simulink model "FPRHX_Demo"  (R2023a)
settings: Solver=FixedStepAuto  StartTime=0.0  StopTime=259200  FixedStep=10  RelTol=1e-3
settings Model: Creator=Owner  LastModifiedBy=Owner

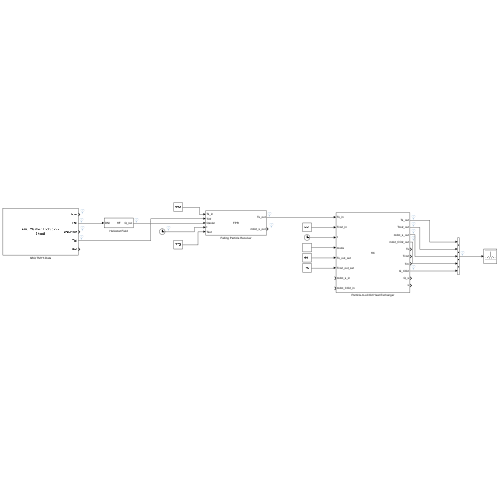
[thumbnail: Simulink's stored preview of the top-level diagram]
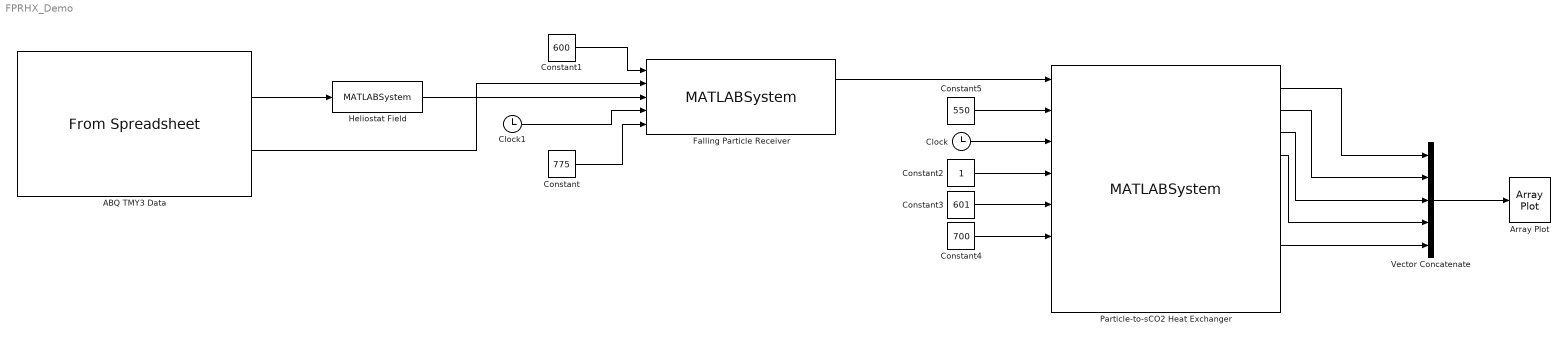
== system FPRHX_Demo ==
  ABQ TMY3 Data : FromSpreadsheet  FileName=ABQ_Weather_Lookup.xlsx  OutDataTypeStr=double
  Array Plot : ArrayPlot  WindowPosition=[1014.000000,178.000000,800.000000,500.000000,]  ScopeFrameLocation=window  YLimits=[-2854873.1962,317687.6016]
  Clock : Clock
  Clock1 : Clock
  Constant : Constant  Value=775
  Constant1 : Constant  Value=600
  Constant2 : Constant  OutDataTypeStr=boolean
  Constant3 : Constant  Value=601
  Constant4 : Constant  Value=700
  Constant5 : Constant  Value=550
  Falling Particle Receiver : MATLABSystem  System=FPR  H=1.2  W=1.2  d=0.0417  SimulateUsing=Code generation  Ts0=600  hInf=5  cp_s=1250  rho_s=3500  phi_s=0.6  epsilon_s=0.88  alpha_s=0.92  tauLag=1500  tauLead=100
      mask Type: FPR
      mask Display:
      | disp('FPR');
      | port_label('input',1,'Ts_in');
      | port_label('input',2,'Tinf');
      | port_label('input',3,'Qsolar');
      | port_label('input',4,'t');
      | port_label('input',5,'Tset');
      | port_label('output',1,'Ts_out');
      | port_label('output',2,'mdot_s_out');
  Heliostat Field : MATLABSystem  System=HF  n=150  H=5  W=5  eta_op=0.6  SimulateUsing=Code generation
      mask Type: HF
      mask Display:
      | disp('HF');
      | port_label('input',1,'DNI');
      | port_label('output',1,'Q_rec');
  Particle-to-sCO2 Heat Exchanger : MATLABSystem  System=HX  n=20  t_s=0.006  t_CO2=0.001  t_m=0.003  H=1.5  W=0.6  N_plate=33  SimulateUsing=Code generation  Ts0=600  Tco20=600  Tm0=25  h_s=450  h_CO2=3000  cp_s=1250  rho_s=3500  phi_s=0.6  cp_CO2=1250  rho_CO2=110  cp_m=500  rho_m=8000
      mask Type: HX
      mask Display:
      | disp('HX');
      | port_label('input',1,'Ts_in');
      | port_label('input',2,'Tco2_in');
      | port_label('input',3,'t');
      | port_label('input',4,'mode');
      | port_label('input',5,'Ts_out_set');
      | port_label('input',6,'Tco2_out_set');
      | port_label('input',7,'mdot_s_in');
      | port_label('input',8,'mdot_CO2_in');
      | port_label('output',1,'Ts_out');
      | port_label('output',2,'Tco2_out');
      | port_label('output',3,'mdot_s_out');
      | port_label('output',4,'mdot_CO2_out');
      | port_label('output',5,'Ts');
      | port_label('output',6,'Tco2');
      | port_label('output',7,'Tm');
      | port_label('output',8,'Q_CO2');
      | port_label('output',9,'Q_s');
      | port_label('output',10,'x');
  Vector Concatenate : Concatenate  NumInputs=5
  wires:
  ABQ TMY3 Data/4 -> Falling Particle Receiver/2
  ABQ TMY3 Data/2 -> Heliostat Field/1
  Clock1/1 -> Falling Particle Receiver/4
  Heliostat Field/1 -> Falling Particle Receiver/3
  Constant1/1 -> Falling Particle Receiver/1
  Constant/1 -> Falling Particle Receiver/5
  Falling Particle Receiver/1 -> Particle-to-sCO2 Heat Exchanger/1
  Constant3/1 -> Particle-to-sCO2 Heat Exchanger/5
  Constant2/1 -> Particle-to-sCO2 Heat Exchanger/4
  Constant4/1 -> Particle-to-sCO2 Heat Exchanger/6
  Constant5/1 -> Particle-to-sCO2 Heat Exchanger/2
  Clock/1 -> Particle-to-sCO2 Heat Exchanger/3
  Particle-to-sCO2 Heat Exchanger/1 -> Vector Concatenate/1
  Particle-to-sCO2 Heat Exchanger/2 -> Vector Concatenate/2
  Particle-to-sCO2 Heat Exchanger/3 -> Vector Concatenate/3
  Particle-to-sCO2 Heat Exchanger/4 -> Vector Concatenate/4
  Particle-to-sCO2 Heat Exchanger/8 -> Vector Concatenate/5
  Vector Concatenate/1 -> Array Plot/1
